simulink subsystem "win_error_decode"  (R2022b)
settings: Solver=VariableStepAuto  StartTime=0.0  StopTime=10.0  RelTol=1e-3
settings Model: Creator=PROSTJP  LastModifiedBy=PROSTJP

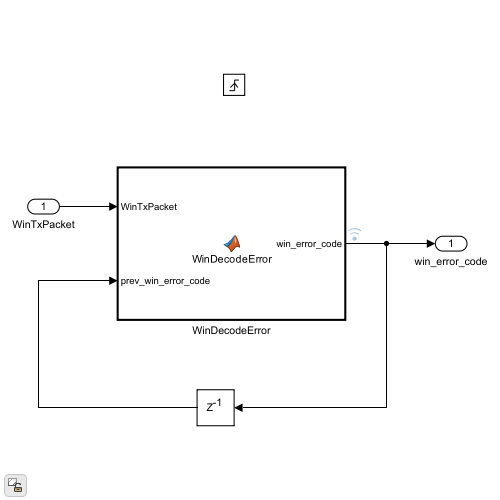
[thumbnail: Simulink's stored preview of the top-level diagram]
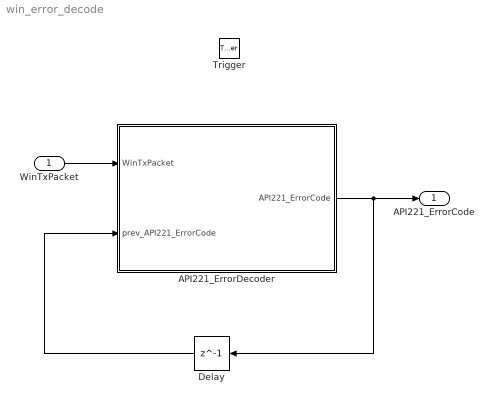
== system win_error_decode ==
  WinTxPacket : Inport
  Trigger : TriggerPort  VariantControl=(inherit)  PortDimensions=1
  API221_ErrorDecoder : MATLAB Function  TreatAsAtomicUnit=on
  Delay : Delay  DelayLength=1
  API221_ErrorCode : Outport
  wires:
  API221_ErrorDecoder/1(API221_ErrorCode) -> API221_ErrorCode/1, Delay/1
  Delay/1 -> API221_ErrorDecoder/2(prev_API221_ErrorCode)
  WinTxPacket/1 -> API221_ErrorDecoder/1(WinTxPacket)

== matlab function win_error_decode/API221_ErrorDecoder ==
  data: WinTxPacket input; API221_ErrorCode output; prev_API221_ErrorCode input double
function API221_ErrorCode = API221_ErrorDecoder(WinTxPacket, prev_API221_ErrorCode)
API221_ErrorCode = prev_API221_ErrorCode;
%if prev_win_error_code == 0
    for i=1:length(WinTxPacket)
        if i < length(WinTxPacket)
            if WinTxPacket(i) == 221 && WinTxPacket(i+1) == 33
                API221_ErrorCode = double(WinTxPacket(i+3))*2^24 + double(WinTxPacket(i+4))*2^16 + double(WinTxPacket(i+5))*2^8 + double(WinTxPacket(i+6));
            end
        end
    end
%else
 %   win_error_code = prev_win_error_code;
%end
